simulink model "example_of_compare_to_zero"  (R2021a)
settings: Solver=VariableStepAuto  StartTime=0.0  StopTime=10  MaxStep=1e-3  RelTol=1e-3
libraries: simulink x3
settings Model: Creator=YasserNet  LastModifiedBy=YasserNet

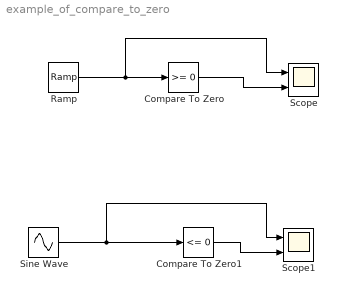
== system example_of_compare_to_zero ==
  Compare To Zero : simulink/Logic and Bit Operations/Compare To Zero  relop=>=  OutDataTypeStr=boolean
  Compare To Zero1 : simulink/Logic and Bit Operations/Compare To Zero  relop=<=  OutDataTypeStr=boolean
  Ramp : simulink/Sources/Ramp  slope=1  start=2  InitialOutput=-0.5
  Scope : Scope  NumInputPorts=2
  Scope1 : Scope  NumInputPorts=2
  Sine Wave : Sin  Frequency=2*pi*3  SampleTime=0
  wires:
  Ramp/1 -> Scope/1, Compare To Zero/1
  Compare To Zero1/1 -> Scope1/2
  Compare To Zero/1 -> Scope/2
  Sine Wave/1 -> Scope1/1, Compare To Zero1/1
